simulink model "Model"  (R2018a)
settings: Solver=VariableStepAuto  StartTime=0.0  StopTime=100  RelTol=1e-3
libraries: simulink_extras x2, templibrary x1
settings Model: Creator=aswerdlow  LastModifiedBy=aswerdlow

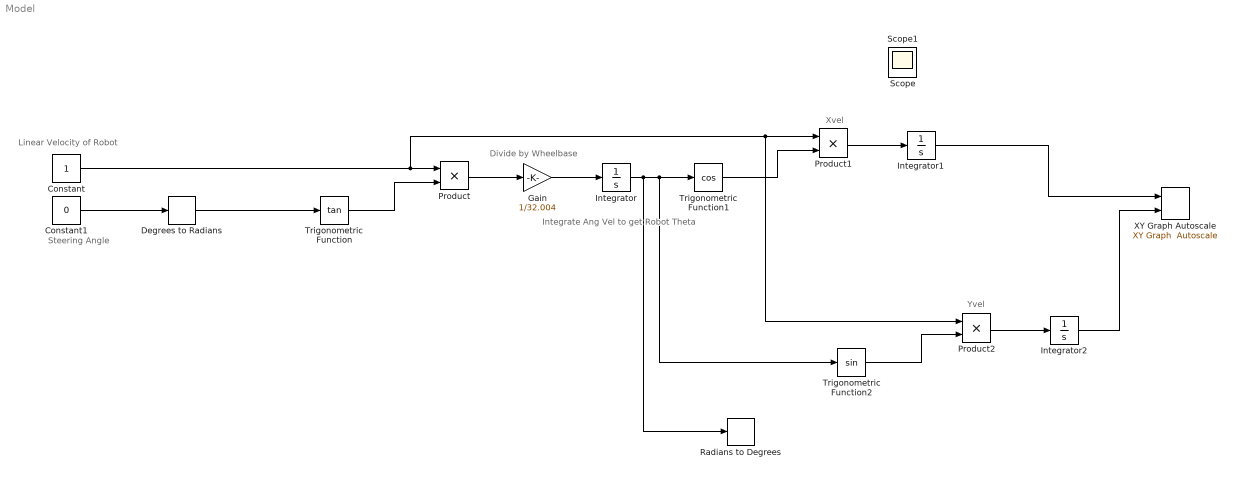
== system Model ==
  note: Yvel
  note: Xvel
  note: Integrate Ang Vel to get Robot Theta
  note: Steering Angle
  note: Linear Velocity of Robot
  note: Divide by Wheelbase
  Constant : Constant
  Constant1 : Constant  Value=0
  Degrees to Radians : simulink_extras/Transformations/Degrees to Radians
  Gain : Gain  Gain=1/32.004
  Integrator : Integrator
  Integrator1 : Integrator
  Integrator2 : Integrator
  Product : Product
  Product1 : Product
  Product2 : Product
  Radians to Degrees : simulink_extras/Transformations/Radians to Degrees
  Trigonometric Function : Trigonometry  Operator=tan
  Trigonometric Function1 : Trigonometry  Operator=cos
  Trigonometric Function2 : Trigonometry
  XY Graph Autoscale : templibrary/XY Graph  Autoscale  xmin=-1  xmax=1  ymin=-1  ymax=1  st=-1
  Scope : Scope
  Scope1 : Scope
  wires:
  Constant/1 -> Product2/1, Product1/1, Product/1
  Constant1/1 -> Degrees to Radians/1
  Degrees to Radians/1 -> Trigonometric Function/1
  Trigonometric Function/1 -> Product/2
  Product/1 -> Gain/1
  Gain/1 -> Integrator/1
  Trigonometric Function1/1 -> Product1/2
  Product1/1 -> Integrator1/1
  Trigonometric Function2/1 -> Product2/2
  Product2/1 -> Integrator2/1
  Integrator/1 -> Radians to Degrees/1, Trigonometric Function2/1, Trigonometric Function1/1
  Integrator1/1 -> XY Graph Autoscale/1
  Integrator2/1 -> XY Graph Autoscale/2
